simulink model "RefModel_rotor"  (R2019b)
settings: Solver=ode1  StartTime=0  StopTime=10  FixedStep=1/sensorFs.imuUpdateFs  RelTol=1e-3
undefined symbols (not defined in the file or in its folder): ACTUATOR_SET
libraries: simulink x1
settings Model: PauseTimes=[10 20]  Creator=sl  LastModifiedBy=sl
settings SolverCC: AutoInsertRateTranBlk=on
settings OptimizationCC: DefaultParameterBehavior=Inlined  EnhancedBackFolding=on  PassReuseOutputArgsAs=Individual arguments  ZeroExternalMemoryAtStartup=off  ZeroInternalMemoryAtStartup=off  MaxStackSize=64  OptimizeBlockOrder=speed  DifferentSizesBufferReuse=on  EfficientTunableParamExpr=on
settings DebuggingCC: MultiTaskCondExecSysMsg=none  ParameterTunabilityLossMsg=error  UnconnectedInputMsg=none  UnconnectedOutputMsg=none  UnconnectedLineMsg=none
settings HardwareCC: ProdBitPerPointer=32  ProdBitPerSizeT=32  ProdBitPerPtrDiffT=32  ProdLargestAtomicInteger=Long  ProdLargestAtomicFloat=Double  ProdWordSize=32  ProdHWDeviceType=ARM Compatible->ARM Cortex
settings SFSimCC: MATLABDynamicMemAlloc=off
settings RTWCC: SystemTargetFile=ert.tlc  TemplateMakefile=ert_default_tmf  GenerateReport=on  Toolchain=GNU Tools for ARM Embedded Processors  IncludeHyperlinkInReport=on  LaunchReport=on  GenerateTraceInfo=on  GenerateTraceReport=on  GenerateTraceReportSl=on  GenerateTraceReportSf=on  GenerateTraceReportEml=on
settings CodeAppCC: ForceParamTrailComments=on  IgnoreCustomStorageClasses=off  OperatorAnnotations=on  SimulinkDataObjDesc=on  SFDataObjDesc=on  InsertBlockDesc=on
settings ERTTargetCC: InlinedParameterPlacement=NonHierarchical  ERTCustomFileTemplate=example_file_process.tlc

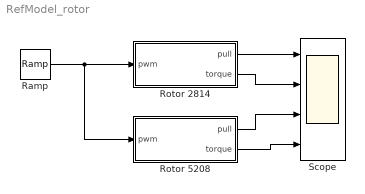
== system RefModel_rotor ==
  Ramp : simulink/Sources/Ramp  slope=100  start=0  InitialOutput=1000
  Rotor 2814 : Subsystem
  Rotor 5208 : Subsystem
  Scope : Scope  NumInputPorts=4
  wires:
  Ramp/1 -> Rotor 5208/1(pwm), Rotor 2814/1(pwm)
  Rotor 2814/1(pull) -> Scope/1
  Rotor 5208/2(torque) -> Scope/4
  Rotor 2814/2(torque) -> Scope/2
  Rotor 5208/1(pull) -> Scope/3

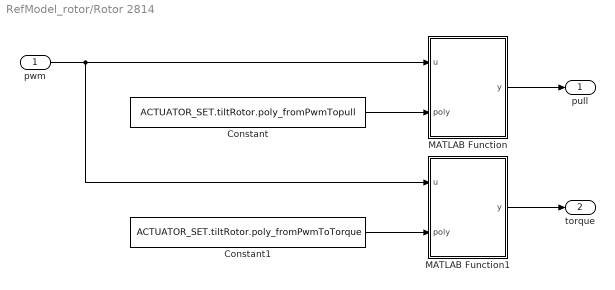
== system RefModel_rotor/Rotor 2814 ==
  pwm : Inport
  Constant : Constant  Value=ACTUATOR_SET.tiltRotor.poly_fromPwmTopull
  Constant1 : Constant  Value=ACTUATOR_SET.tiltRotor.poly_fromPwmToTorque
  MATLAB Function : MATLAB Function  TreatAsAtomicUnit=on
  MATLAB Function1 : MATLAB Function  TreatAsAtomicUnit=on
  pull : Outport
  torque : Outport  Port=2
  wires:
  pwm/1 -> MATLAB Function1/1(u), MATLAB Function/1(u)
  MATLAB Function/1(y) -> pull/1
  Constant/1 -> MATLAB Function/2(poly)
  Constant1/1 -> MATLAB Function1/2(poly)
  MATLAB Function1/1(y) -> torque/1

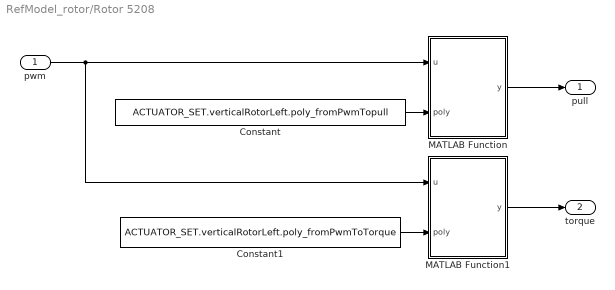
== system RefModel_rotor/Rotor 5208 ==
  pwm : Inport
  Constant : Constant  Value=ACTUATOR_SET.verticalRotorLeft.poly_fromPwmTopull
  Constant1 : Constant  Value=ACTUATOR_SET.verticalRotorLeft.poly_fromPwmToTorque
  MATLAB Function : MATLAB Function  TreatAsAtomicUnit=on
  MATLAB Function1 : MATLAB Function  TreatAsAtomicUnit=on
  pull : Outport
  torque : Outport  Port=2
  wires:
  MATLAB Function1/1(y) -> torque/1
  Constant1/1 -> MATLAB Function1/2(poly)
  Constant/1 -> MATLAB Function/2(poly)
  MATLAB Function/1(y) -> pull/1
  pwm/1 -> MATLAB Function/1(u), MATLAB Function1/1(u)

== matlab function RefModel_rotor/Rotor 2814/MATLAB Function1 ==
  data: u input; y output; poly input
function y = fcn(u, poly)
vec = [u^2,u,1];
y = dot(vec,poly);

== matlab function RefModel_rotor/Rotor 2814/MATLAB Function ==
  data: u input; y output; poly input
function y = fcn(u, poly)
vec = [u^2,u,1];
y = dot(vec,poly);

== matlab function RefModel_rotor/Rotor 5208/MATLAB Function ==
  data: u input; y output; poly input
function y = fcn(u, poly)
vec = [u^2,u,1];
y = dot(vec,poly);

== matlab function RefModel_rotor/Rotor 5208/MATLAB Function1 ==
  data: u input; y output; poly input
function y = fcn(u, poly)
vec = [u^2,u,1];
y = dot(vec,poly);
